simulink library "Dynamics_and_Kinematics"  (R2022b)
settings: Solver=VariableStepAuto  StartTime=0.0  StopTime=10.0  RelTol=1e-3
undefined symbols (not defined in the file): Config
libraries: WBToolboxLibrary x21
settings Model: Creator=fdinatale  LastModifiedBy=fdinatale

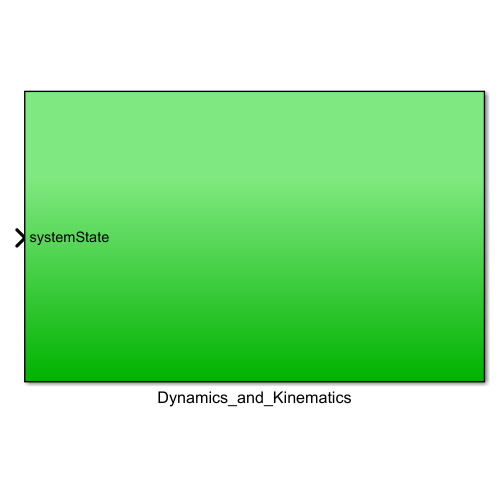
[thumbnail: Simulink's stored preview of the top-level diagram]
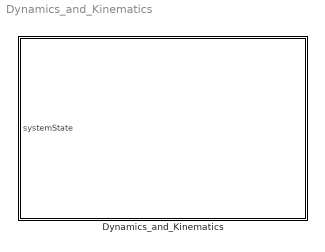
== system Dynamics_and_Kinematics ==
  Dynamics_and_Kinematics : Subsystem

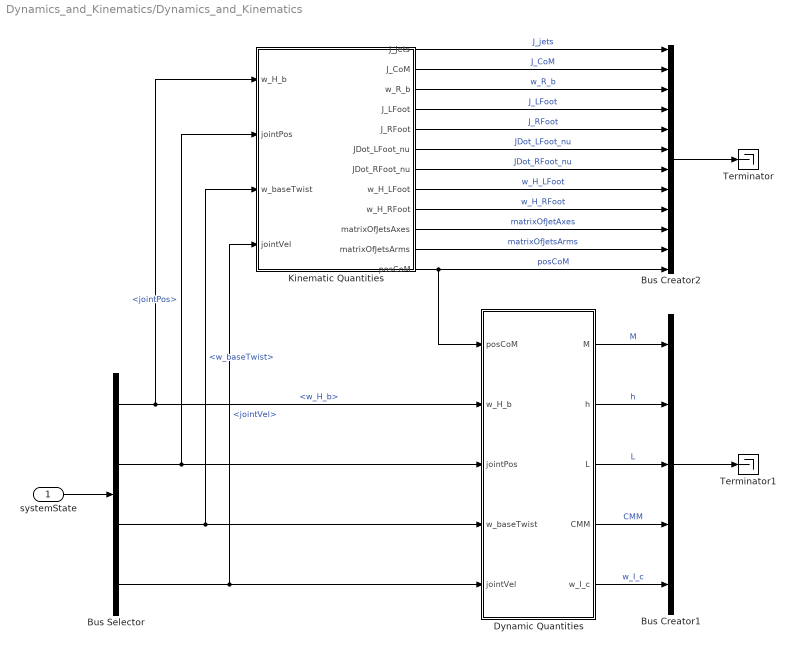
== system Dynamics_and_Kinematics/Dynamics_and_Kinematics ==
  systemState : Inport
  Bus Creator1 : BusCreator  Inputs=5
  Bus Creator2 : BusCreator  Inputs=12
  Bus Selector : BusSelector  OutputSignals=w_H_b,jointPos,w_baseTwist,jointVel
  Dynamic Quantities : Subsystem
  Kinematic Quantities : Subsystem
  Terminator : Terminator
  Terminator1 : Terminator
  wires:
  Kinematic Quantities/2(J_CoM) -> Bus Creator2/2  "J_CoM"
  Bus Creator1/1 -> Terminator1/1
  Bus Selector/2 -> Kinematic Quantities/2(jointPos), Dynamic Quantities/3(jointPos)  "<jointPos>"
  Bus Selector/1 -> Kinematic Quantities/1(w_H_b), Dynamic Quantities/2(w_H_b)  "<w_H_b>"
  Kinematic Quantities/6(JDot_LFoot_nu) -> Bus Creator2/6  "JDot_LFoot_nu"
  Dynamic Quantities/4(CMM) -> Bus Creator1/4  "CMM"
  Kinematic Quantities/12(posCoM) -> Dynamic Quantities/1(posCoM), Bus Creator2/12  "posCoM"
  Kinematic Quantities/8(w_H_LFoot) -> Bus Creator2/8  "w_H_LFoot"
  Bus Creator2/1 -> Terminator/1
  Kinematic Quantities/11(matrixOfJetsArms) -> Bus Creator2/11  "matrixOfJetsArms"
  Bus Selector/4 -> Kinematic Quantities/4(jointVel), Dynamic Quantities/5(jointVel)  "<jointVel>"
  Kinematic Quantities/1(J_jets) -> Bus Creator2/1  "J_jets"
  Kinematic Quantities/3(w_R_b) -> Bus Creator2/3  "w_R_b"
  Dynamic Quantities/2("h ") -> Bus Creator1/2  "h"
  Dynamic Quantities/3(L) -> Bus Creator1/3  "L"
  Bus Selector/3 -> Kinematic Quantities/3(w_baseTwist), Dynamic Quantities/4(w_baseTwist)  "<w_baseTwist>"
  Kinematic Quantities/5(J_RFoot) -> Bus Creator2/5  "J_RFoot"
  Kinematic Quantities/9(w_H_RFoot) -> Bus Creator2/9  "w_H_RFoot"
  Kinematic Quantities/4(J_LFoot) -> Bus Creator2/4  "J_LFoot"
  Kinematic Quantities/10(matrixOfJetsAxes) -> Bus Creator2/10  "matrixOfJetAxes"
  Dynamic Quantities/5(w_I_c) -> Bus Creator1/5  "w_I_c"
  systemState/1 -> Bus Selector/1
  Kinematic Quantities/7(JDot_RFoot_nu) -> Bus Creator2/7  "JDot_RFoot_nu"
  Dynamic Quantities/1(M) -> Bus Creator1/1  "M"

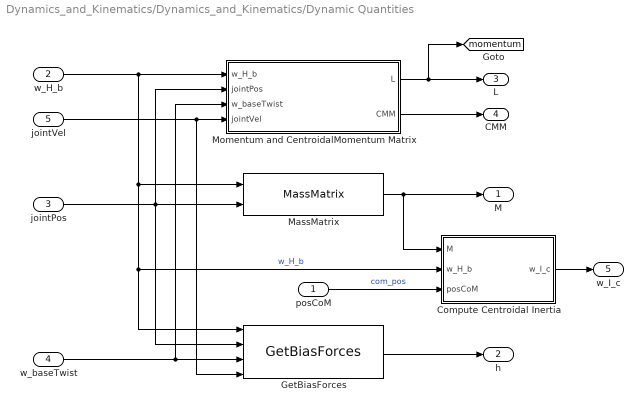
== system Dynamics_and_Kinematics/Dynamics_and_Kinematics/Dynamic Quantities ==
  posCoM : Inport
  w_H_b : Inport  Port=2
  jointPos : Inport  Port=3
  w_baseTwist : Inport  Port=4
  jointVel : Inport  Port=5
  Compute Centroidal Inertia : Subsystem
  GetBiasForces : WBToolboxLibrary/Model/Dynamics/GetBiasForces
      settings: SourceProductName=WholeBodyToolbox
  MassMatrix : WBToolboxLibrary/Model/Dynamics/MassMatrix
      settings: SourceProductName=WholeBodyToolbox
  Momentum and CentroidalMomentum Matrix : Subsystem
  M : Outport  VectorParamsAs1DForOutWhenUnconnected=off
  "h " : Outport  Port=2  VectorParamsAs1DForOutWhenUnconnected=off
  L : Outport  Port=3  VectorParamsAs1DForOutWhenUnconnected=off
  CMM : Outport  Port=4  VectorParamsAs1DForOutWhenUnconnected=off
  w_I_c : Outport  Port=5  VectorParamsAs1DForOutWhenUnconnected=off
  tag scope: momentum=global
  wires:
  posCoM/1 -> Compute Centroidal Inertia/3(posCoM)  "com_pos"
  Compute Centroidal Inertia/1(w_I_c) -> w_I_c/1
  jointPos/1 -> Momentum and CentroidalMomentum Matrix/2(jointPos), MassMatrix/2, GetBiasForces/2
  Momentum and CentroidalMomentum Matrix/1(L) -> [momentum], L/1
  Momentum and CentroidalMomentum Matrix/2(CMM) -> CMM/1
  GetBiasForces/1 -> "h "/1
  MassMatrix/1 -> M/1, Compute Centroidal Inertia/1(M)
  jointVel/1 -> GetBiasForces/4, Momentum and CentroidalMomentum Matrix/4(jointVel)
  w_baseTwist/1 -> GetBiasForces/3, Momentum and CentroidalMomentum Matrix/3(w_baseTwist)
  w_H_b/1 -> MassMatrix/1, Compute Centroidal Inertia/2(w_H_b), GetBiasForces/1, Momentum and CentroidalMomentum Matrix/1(w_H_b)  "w_H_b"

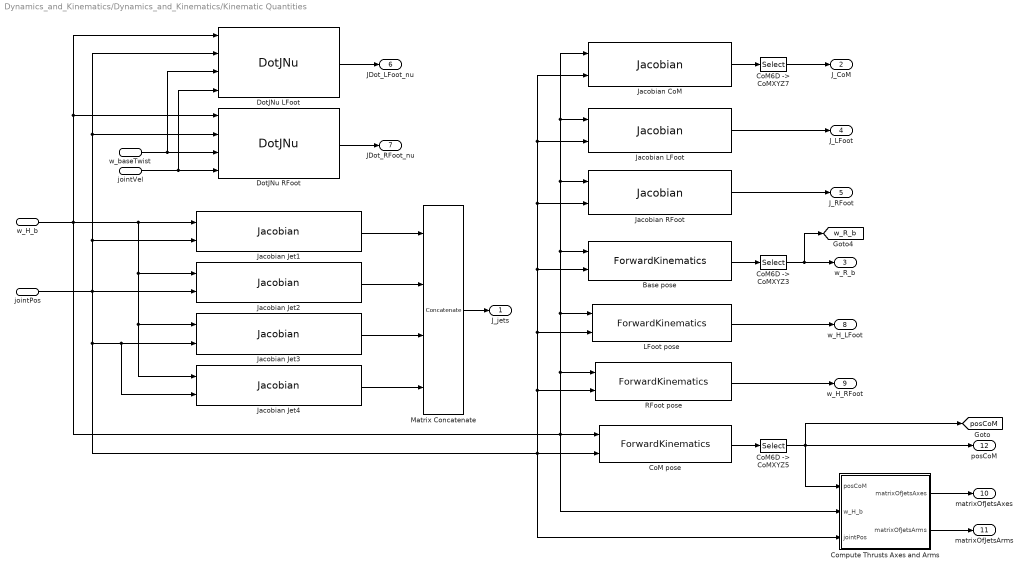
== system Dynamics_and_Kinematics/Dynamics_and_Kinematics/Kinematic Quantities ==
  w_H_b : Inport
  jointPos : Inport  Port=2
  w_baseTwist : Inport  Port=3
  jointVel : Inport  Port=4
  Base pose : WBToolboxLibrary/Model/Kinematics/ForwardKinematics  frameName=Frames.BASE_LINK
      settings: SourceProductName=WholeBodyToolbox
  CoM pose : WBToolboxLibrary/Model/Kinematics/ForwardKinematics  frameName=Frames.COM_FRAME
      settings: SourceProductName=WholeBodyToolbox
  "CoM6D -> CoMXYZ3" : Selector  NumberOfDimensions=2  InputPortWidth=7  IndexOptions=Index vector (dialog),Index vector (dialog)  Indices=[1 2 3],[1 2 3]  OutputSizes=1,1
  "CoM6D -> CoMXYZ5" : Selector  NumberOfDimensions=2  InputPortWidth=7  IndexOptions=Index vector (dialog),Index vector (dialog)  Indices=[1 2 3],[4]  OutputSizes=1,1
  "CoM6D -> CoMXYZ7" : Selector  NumberOfDimensions=2  InputPortWidth=7  IndexOptions=Index vector (dialog),Index vector (dialog)  Indices=[1 2 3],[1:6+Config.N_DOF]  OutputSizes=1,1
  Compute Thrusts Axes and Arms : Subsystem
  DotJNu LFoot : WBToolboxLibrary/Model/Jacobians/DotJNu  frameName=Frames.LFOOT_FRAME
      settings: SourceProductName=WholeBodyToolbox
  DotJNu RFoot : WBToolboxLibrary/Model/Jacobians/DotJNu  frameName=Frames.RFOOT_FRAME
      settings: SourceProductName=WholeBodyToolbox
  Jacobian CoM : WBToolboxLibrary/Model/Jacobians/Jacobian  frameName=Frames.COM_FRAME
      settings: SourceProductName=WholeBodyToolbox
  Jacobian Jet1 : WBToolboxLibrary/Model/Jacobians/Jacobian  frameName=Frames.JET1_FRAME
      settings: SourceProductName=WholeBodyToolbox
  Jacobian Jet2 : WBToolboxLibrary/Model/Jacobians/Jacobian  frameName=Frames.JET2_FRAME
      settings: SourceProductName=WholeBodyToolbox
  Jacobian Jet3 : WBToolboxLibrary/Model/Jacobians/Jacobian  frameName=Frames.JET3_FRAME
      settings: SourceProductName=WholeBodyToolbox
  Jacobian Jet4 : WBToolboxLibrary/Model/Jacobians/Jacobian  frameName=Frames.JET4_FRAME
      settings: SourceProductName=WholeBodyToolbox
  Jacobian LFoot : WBToolboxLibrary/Model/Jacobians/Jacobian  frameName=Frames.LFOOT_FRAME
      settings: SourceProductName=WholeBodyToolbox
  Jacobian RFoot : WBToolboxLibrary/Model/Jacobians/Jacobian  frameName=Frames.RFOOT_FRAME
      settings: SourceProductName=WholeBodyToolbox
  LFoot pose : WBToolboxLibrary/Model/Kinematics/ForwardKinematics  frameName=Frames.LFOOT_FRAME
      settings: SourceProductName=WholeBodyToolbox
  Matrix Concatenate : Concatenate  NumInputs=4  Mode=Multidimensional array
  RFoot pose : WBToolboxLibrary/Model/Kinematics/ForwardKinematics  frameName=Frames.RFOOT_FRAME
      settings: SourceProductName=WholeBodyToolbox
  J_jets : Outport  VectorParamsAs1DForOutWhenUnconnected=off
  J_CoM : Outport  Port=2  VectorParamsAs1DForOutWhenUnconnected=off
  w_R_b : Outport  Port=3  VectorParamsAs1DForOutWhenUnconnected=off
  J_LFoot : Outport  Port=4  VectorParamsAs1DForOutWhenUnconnected=off
  J_RFoot : Outport  Port=5  VectorParamsAs1DForOutWhenUnconnected=off
  JDot_LFoot_nu : Outport  Port=6  VectorParamsAs1DForOutWhenUnconnected=off
  JDot_RFoot_nu : Outport  Port=7  VectorParamsAs1DForOutWhenUnconnected=off
  w_H_LFoot : Outport  Port=8  VectorParamsAs1DForOutWhenUnconnected=off
  w_H_RFoot : Outport  Port=9  VectorParamsAs1DForOutWhenUnconnected=off
  matrixOfJetsAxes : Outport  Port=10  VectorParamsAs1DForOutWhenUnconnected=off
  matrixOfJetsArms : Outport  Port=11  VectorParamsAs1DForOutWhenUnconnected=off
  posCoM : Outport  Port=12  VectorParamsAs1DForOutWhenUnconnected=off
  tag scope: posCoM=global, w_R_b=global
  wires:
  "CoM6D -> CoMXYZ7"/1 -> J_CoM/1
  Jacobian Jet4/1 -> Matrix Concatenate/4
  Jacobian Jet3/1 -> Matrix Concatenate/3
  Jacobian Jet2/1 -> Matrix Concatenate/2
  Jacobian Jet1/1 -> Matrix Concatenate/1
  Compute Thrusts Axes and Arms/1(matrixOfJetsAxes) -> matrixOfJetsAxes/1
  Compute Thrusts Axes and Arms/2(matrixOfJetsArms) -> matrixOfJetsArms/1
  Base pose/1 -> "CoM6D -> CoMXYZ3"/1
  LFoot pose/1 -> w_H_LFoot/1
  RFoot pose/1 -> w_H_RFoot/1
  w_baseTwist/1 -> DotJNu RFoot/3, DotJNu LFoot/3
  jointVel/1 -> DotJNu LFoot/4, DotJNu RFoot/4
  DotJNu LFoot/1 -> JDot_LFoot_nu/1
  DotJNu RFoot/1 -> JDot_RFoot_nu/1
  Jacobian LFoot/1 -> J_LFoot/1
  Jacobian RFoot/1 -> J_RFoot/1
  Jacobian CoM/1 -> "CoM6D -> CoMXYZ7"/1
  jointPos/1 -> Jacobian Jet1/2, DotJNu RFoot/2, DotJNu LFoot/2, Jacobian Jet2/2, CoM pose/2, RFoot pose/2, Base pose/2, Jacobian CoM/2, Jacobian LFoot/2, Jacobian RFoot/2, LFoot pose/2, Compute Thrusts Axes and Arms/3(jointPos), Jacobian Jet3/2, Jacobian Jet4/2
  "CoM6D -> CoMXYZ3"/1 -> [w_R_b], w_R_b/1
  w_H_b/1 -> Jacobian Jet1/1, Jacobian Jet2/1, Jacobian Jet3/1, Jacobian Jet4/1, DotJNu RFoot/1, DotJNu LFoot/1, Compute Thrusts Axes and Arms/2(w_H_b), CoM pose/1, RFoot pose/1, Jacobian RFoot/1, Jacobian CoM/1, Jacobian LFoot/1, Base pose/1, LFoot pose/1
  "CoM6D -> CoMXYZ5"/1 -> Compute Thrusts Axes and Arms/1(posCoM), [posCoM], posCoM/1
  CoM pose/1 -> "CoM6D -> CoMXYZ5"/1
  Matrix Concatenate/1 -> J_jets/1

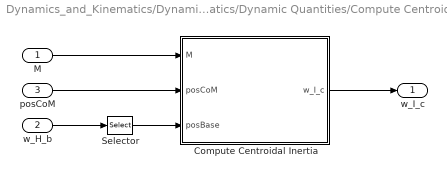
== system Dynamics_and_Kinematics/Dynamics_and_Kinematics/Dynamic Quantities/Compute Centroidal Inertia ==
  M : Inport
  w_H_b : Inport  Port=2
  posCoM : Inport  Port=3
  Compute Centroidal Inertia : MATLAB Function  TreatAsAtomicUnit=on
  Selector : Selector  NumberOfDimensions=2  InputPortWidth=3  IndexOptions=Index vector (dialog),Index vector (dialog)  Indices=[1 2 3],4  OutputSizes=1,1
  w_I_c : Outport  VectorParamsAs1DForOutWhenUnconnected=off
  wires:
  Compute Centroidal Inertia/1(w_I_c) -> w_I_c/1
  posCoM/1 -> Compute Centroidal Inertia/2(posCoM)
  Selector/1 -> Compute Centroidal Inertia/3(posBase)
  w_H_b/1 -> Selector/1
  M/1 -> Compute Centroidal Inertia/1(M)

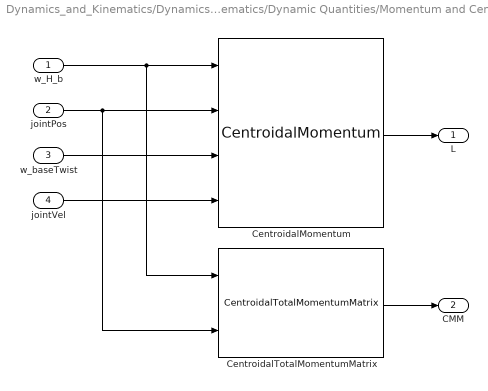
== system Dynamics_and_Kinematics/Dynamics_and_Kinematics/Dynamic Quantities/Momentum and CentroidalMomentum Matrix ==
  w_H_b : Inport
  jointPos : Inport  Port=2
  w_baseTwist : Inport  Port=3
  jointVel : Inport  Port=4
  CentroidalMomentum : WBToolboxLibrary/Model/Dynamics/CentroidalMomentum
      settings: SourceProductName=WholeBodyToolbox
  CentroidalTotalMomentumMatrix : WBToolboxLibrary/Model/Jacobians/CentroidalTotalMomentumMatrix
      settings: SourceProductName=WholeBodyToolbox
  L : Outport  VectorParamsAs1DForOutWhenUnconnected=off
  CMM : Outport  Port=2  VectorParamsAs1DForOutWhenUnconnected=off
  wires:
  CentroidalTotalMomentumMatrix/1 -> CMM/1
  jointVel/1 -> CentroidalMomentum/4
  jointPos/1 -> CentroidalMomentum/2, CentroidalTotalMomentumMatrix/2
  w_H_b/1 -> CentroidalMomentum/1, CentroidalTotalMomentumMatrix/1
  CentroidalMomentum/1 -> L/1
  w_baseTwist/1 -> CentroidalMomentum/3

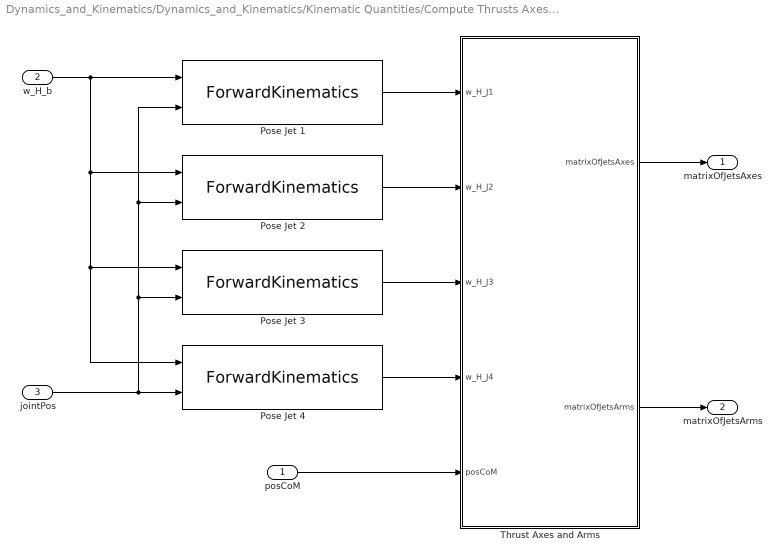
== system Dynamics_and_Kinematics/Dynamics_and_Kinematics/Kinematic Quantities/Compute Thrusts Axes and Arms ==
  posCoM : Inport
  w_H_b : Inport  Port=2
  jointPos : Inport  Port=3
  Pose Jet 1 : WBToolboxLibrary/Model/Kinematics/ForwardKinematics  frameName=Frames.JET1_FRAME
      settings: SourceProductName=WholeBodyToolbox
  Pose Jet 2 : WBToolboxLibrary/Model/Kinematics/ForwardKinematics  frameName=Frames.JET2_FRAME
      settings: SourceProductName=WholeBodyToolbox
  Pose Jet 3 : WBToolboxLibrary/Model/Kinematics/ForwardKinematics  frameName=Frames.JET3_FRAME
      settings: SourceProductName=WholeBodyToolbox
  Pose Jet 4 : WBToolboxLibrary/Model/Kinematics/ForwardKinematics  frameName=Frames.JET4_FRAME
      settings: SourceProductName=WholeBodyToolbox
  Thrust Axes and Arms : MATLAB Function  TreatAsAtomicUnit=on
  matrixOfJetsAxes : Outport  VectorParamsAs1DForOutWhenUnconnected=off
  matrixOfJetsArms : Outport  Port=2  VectorParamsAs1DForOutWhenUnconnected=off
  wires:
  posCoM/1 -> Thrust Axes and Arms/5(posCoM)
  w_H_b/1 -> Pose Jet 1/1, Pose Jet 2/1, Pose Jet 3/1, Pose Jet 4/1
  Thrust Axes and Arms/2(matrixOfJetsArms) -> matrixOfJetsArms/1
  Thrust Axes and Arms/1(matrixOfJetsAxes) -> matrixOfJetsAxes/1
  Pose Jet 4/1 -> Thrust Axes and Arms/4(w_H_J4)
  Pose Jet 3/1 -> Thrust Axes and Arms/3(w_H_J3)
  Pose Jet 1/1 -> Thrust Axes and Arms/1(w_H_J1)
  jointPos/1 -> Pose Jet 4/2, Pose Jet 3/2, Pose Jet 2/2, Pose Jet 1/2
  Pose Jet 2/1 -> Thrust Axes and Arms/2(w_H_J2)

== matlab function Dynamics_and_Kinematics/Kinematic Quantities/Compute Thrusts Axes and Arms/Thrust Axes and Arms ==
  data: w_H_J1 input; matrixOfJetsAxes output; w_H_J2 input; w_H_J3 input; w_H_J4 input; posCoM input; matrixOfJetsArms output; Config parameter
function [matrixOfJetsAxes, matrixOfJetsArms] = computeJetsAxesAndArmsFCN(w_H_J1, w_H_J2, w_H_J3, w_H_J4, posCoM, Config)

    [matrixOfJetsAxes, matrixOfJetsArms] = iRonCubLib.computeJetsAxesAndArms(w_H_J1, w_H_J2, w_H_J3, w_H_J4, posCoM, Config);
end

== matlab function Dynamics_and_Kinematics/Dynamic Quantities/Compute Centroidal Inertia/Compute Centroidal Inertia ==
  data: M input; w_I_c output; posCoM input; posBase input
function w_I_c = getCentrInertiaFCN(M, posCoM, posBase)

    w_I_c = iRonCubLib.getCentrInertia(M, posCoM, posBase);
end
